simulink model "ex1_b"  (R2021b)
settings: Solver=VariableStepAuto  StartTime=0.0  StopTime=10.0  RelTol=1e-3

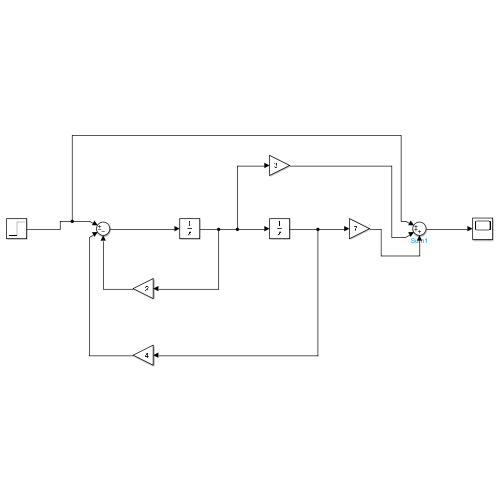
[thumbnail: Simulink's stored preview of the top-level diagram]
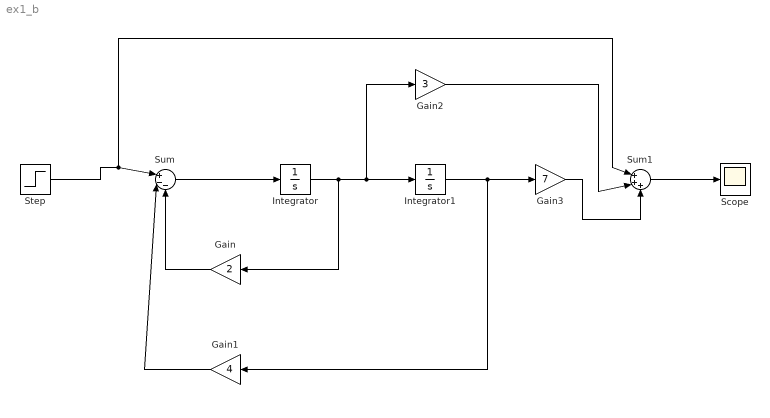
== system ex1_b ==
  Gain : Gain  Gain=2
  Gain1 : Gain  Gain=4
  Gain2 : Gain  Gain=3
  Gain3 : Gain  Gain=7
  Integrator : Integrator
  Integrator1 : Integrator
  Scope : Scope
  Step : Step  SampleTime=0
  Sum : Sum  Inputs=|+--
  Sum1 : Sum  Inputs=|+++
  wires:
  Step/1 -> Sum1/1, Sum/1
  Sum/1 -> Integrator/1
  Integrator/1 -> Gain/1, Gain2/1, Integrator1/1
  Integrator1/1 -> Gain1/1, Gain3/1
  Gain2/1 -> Sum1/2
  Gain3/1 -> Sum1/3
  Sum1/1 -> Scope/1
  Gain/1 -> Sum/3
  Gain1/1 -> Sum/2
